simulink model "two_tanks_PID"  (R2018b)
settings: Solver=FixedStepAuto  StartTime=0.0  StopTime=120  FixedStep=0.1  RelTol=1e-3
model workspace (MATLAB code in the model file):
  | A1 = 1;
  | a1 = 0.1*0.1;
  | A2 = A1;
  | a2 = a1;
  | h10 = 1;
  | h20=1;
libraries: simulink x1
settings Model: EnablePacing=on  PacingRate=5  Creator=kjartan  LastModifiedBy=kjartan

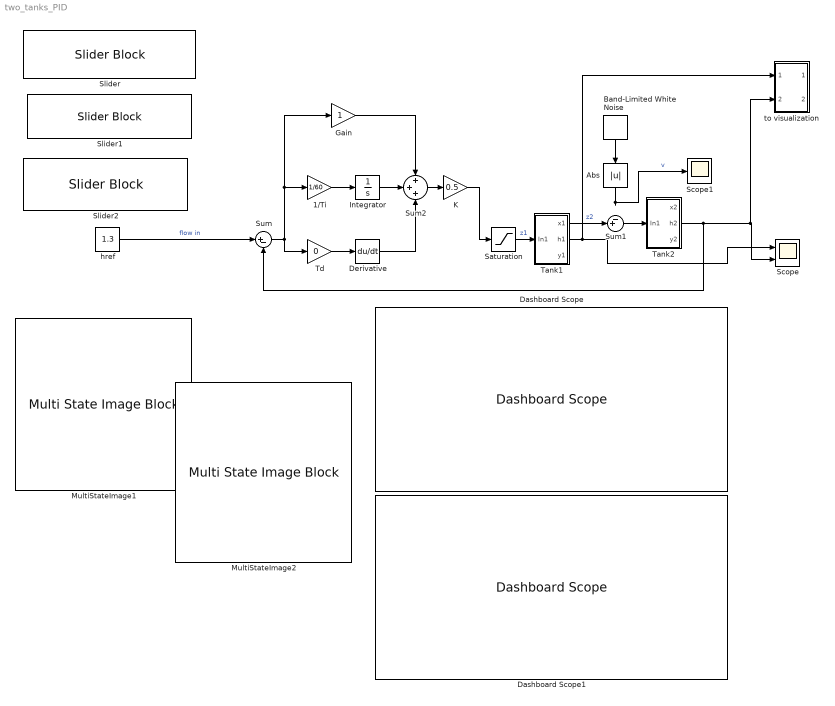
== system two_tanks_PID ==
  1/Ti : Gain  Gain=1/60
  Abs : Abs
  Band-Limited White Noise : simulink/Sources/Band-Limited White Noise  Cov=0.01*0.01  Ts=3  seed=[23341]
  Dashboard Scope : DashboardScope  WebBlockId=50  Ymin=0  Ymax=2.6000000000000001
  Dashboard Scope1 : DashboardScope  WebBlockId=91  Ymin=0  Ymax=0.29999999999999999
  Derivative : Derivative  CoefficientInTFapproximation=100
  Gain : Gain
  Integrator : Integrator
  K : Gain  Gain=0.5
  MultiStateImage1 : MultiStateImageBlock  WebBlockId=71
  MultiStateImage2 : MultiStateImageBlock  WebBlockId=74
  Saturation : Saturate  LowerLimit=0
  Scope : Scope  NumInputPorts=2
  Scope1 : Scope
  Slider : SliderBlock  WebBlockId=82  ScaleMax=0.5
  Slider1 : SliderBlock  WebBlockId=85  ScaleMax=0.10000000000000001
  Slider2 : SliderBlock  WebBlockId=90  ScaleMax=60
  Sum : Sum  Inputs=|+-
  Sum1 : Sum  Inputs=-+|
  Sum2 : Sum  Inputs=+++
  Tank1 : Subsystem
  Tank2 : Subsystem
  Td : Gain  Gain=0
  href : Constant  Value=1.3
  to visualization : Subsystem
  wires:
  Tank1/1(x1) -> Sum1/2  "z2"
  Tank1/2(h1) -> to visualization/1(In2), Scope/1
  Tank2/2(h2) -> to visualization/2(In1), Scope/2, Sum/2
  Sum1/1 -> Tank2/1(In1)
  Band-Limited White Noise/1 -> Abs/1
  Abs/1 -> Scope1/1  "v"
  href/1 -> Sum/1  "flow in"
  Sum/1 -> Td/1, 1/Ti/1, Gain/1
  Derivative/1 -> Sum2/3
  Integrator/1 -> Sum2/2
  Gain/1 -> Sum2/1
  Sum2/1 -> K/1
  1/Ti/1 -> Integrator/1
  Td/1 -> Derivative/1
  Saturation/1 -> Tank1/1(In1)  "z1"
  K/1 -> Saturation/1

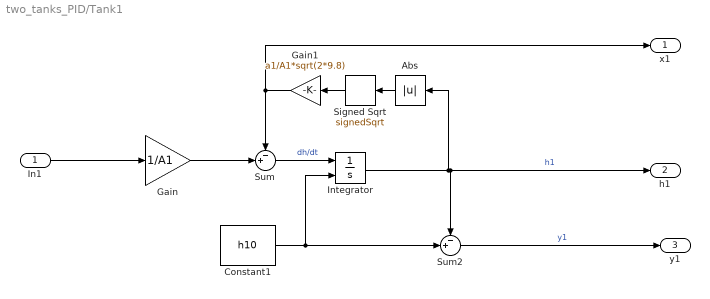
== system two_tanks_PID/Tank1 ==
  In1 : Inport
  Abs : Abs
  Constant1 : Constant  Value=h10
  Gain : Gain  Gain=1/A1
  Gain1 : Gain  Gain=a1/A1*sqrt(2*9.8)
  Integrator : Integrator  InitialConditionSource=external  InitialCondition=h10
  Signed Sqrt : Sqrt  Operator=signedSqrt  SaturateOnIntegerOverflow=on
  Sum : Sum  Inputs=-+|
  Sum2 : Sum  Inputs=-+|
  x1 : Outport
  h1 : Outport  Port=2
  y1 : Outport  Port=3
  wires:
  Gain1/1 -> x1/1, Sum/1
  Gain/1 -> Sum/2
  Sum/1 -> Integrator/1  "dh/dt"
  In1/1 -> Gain/1
  Sum2/1 -> y1/1  "y1"
  Signed Sqrt/1 -> Gain1/1
  Integrator/1 -> h1/1, Sum2/1, Abs/1  "h1"
  Abs/1 -> Signed Sqrt/1
  Constant1/1 -> Sum2/2, Integrator/2

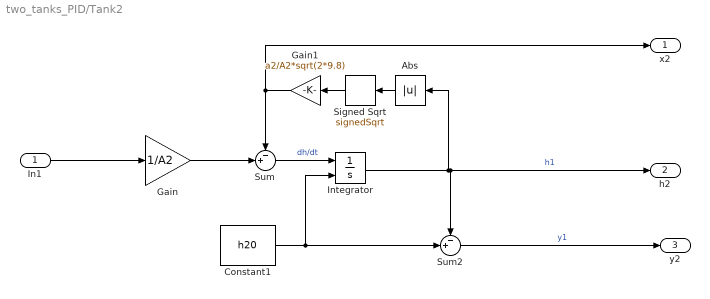
== system two_tanks_PID/Tank2 ==
  In1 : Inport
  Abs : Abs
  Constant1 : Constant  Value=h20
  Gain : Gain  Gain=1/A2
  Gain1 : Gain  Gain=a2/A2*sqrt(2*9.8)
  Integrator : Integrator  InitialConditionSource=external  InitialCondition=h10
  Signed Sqrt : Sqrt  Operator=signedSqrt  SaturateOnIntegerOverflow=on
  Sum : Sum  Inputs=-+|
  Sum2 : Sum  Inputs=-+|
  x2 : Outport
  h2 : Outport  Port=2
  y2 : Outport  Port=3
  wires:
  Gain1/1 -> x2/1, Sum/1
  Gain/1 -> Sum/2
  Sum/1 -> Integrator/1  "dh/dt"
  In1/1 -> Gain/1
  Sum2/1 -> y2/1  "y1"
  Signed Sqrt/1 -> Gain1/1
  Integrator/1 -> h2/1, Sum2/1, Abs/1  "h1"
  Abs/1 -> Signed Sqrt/1
  Constant1/1 -> Sum2/2, Integrator/2

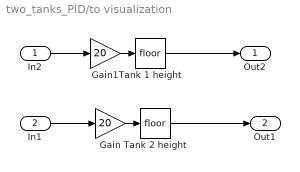
== system two_tanks_PID/to visualization ==
  In2 : Inport
  In1 : Inport  Port=2
  Gain : Gain  Gain=20
  Gain1 : Gain  Gain=20
  Tank 1 height : Rounding
  Tank 2 height : Rounding
  Out2 : Outport
  Out1 : Outport  Port=2
  wires:
  Tank 2 height/1 -> Out1/1
  Gain/1 -> Tank 2 height/1
  In1/1 -> Gain/1
  Tank 1 height/1 -> Out2/1
  Gain1/1 -> Tank 1 height/1
  In2/1 -> Gain1/1
